simulink model "czasRegulacji_uchyb_przeregulowanie_simulink"  (R2025b)
settings: Solver=VariableStepAuto  StartTime=0.0  StopTime=20  RelTol=1e-3
settings Model: Creator=mefir  LastModifiedBy=mefir

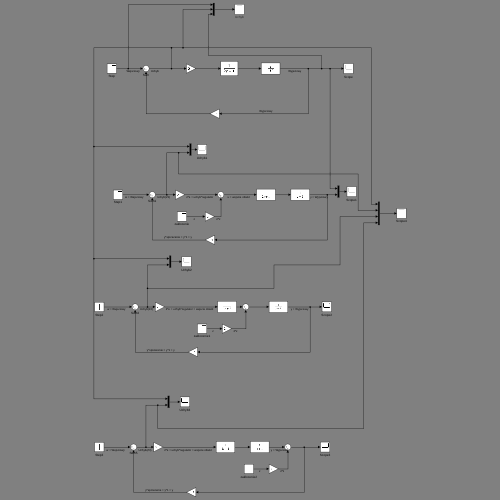
[thumbnail: Simulink's stored preview of the top-level diagram]
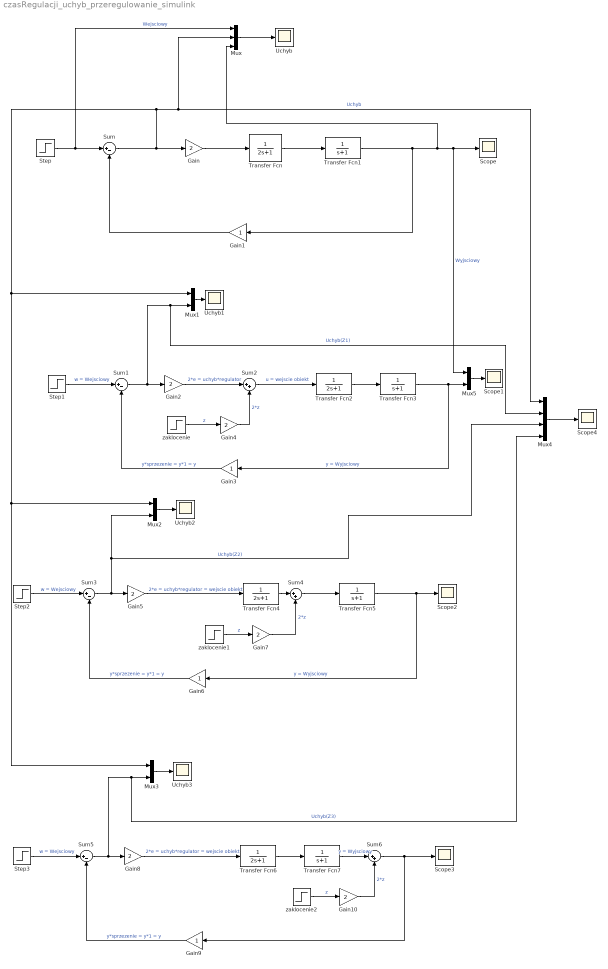
== system czasRegulacji_uchyb_przeregulowanie_simulink ==
  Gain{,2,4..5,7..8,10} (7 alike) : Gain  Gain=2
  Gain{1,3,6,9} (4 alike) : Gain
  Mux : Mux  Inputs=3
  Mux{1..3,5} (4 alike) : Mux  Inputs=2
  Mux4 : Mux
  Scope{,1..4} (5 alike) : Scope
      Scope settings: ActiveDisplayYMinimum=-0.06502980968093075  ActiveDisplayYMaximum=0.77577049871628523
      Scope1 settings: ActiveDisplayYMinimum=-0.023285806575956025  ActiveDisplayYMaximum=2.011000432811886  DataLoggingVariableName=ScopeData2
      Scope2 settings: ActiveDisplayYMinimum=-0.48841878311873588  ActiveDisplayYMaximum=2.237719338068338  DataLoggingVariableName=ScopeData4
      Scope3 settings: ActiveDisplayYMinimum=-0.61690021233914671  ActiveDisplayYMaximum=2.3886670662696021  DataLoggingVariableName=ScopeData6
      Scope4 settings: ActiveDisplayYMinimum=-1.25  ActiveDisplayYMaximum=1.25  DataLoggingVariableName=ScopeData8
  Step{,1..3} (4 alike) : Step  Time=0  SampleTime=0
  Sum{,1,3,5} (4 alike) : Sum  Inputs=|+-
  Sum2 : Sum  Inputs=|++
  Sum4 : Sum  Inputs=|++
  Sum6 : Sum  Inputs=|++
  Transfer Fcn{,2,4,6} (4 alike) : TransferFcn  Denominator=[2 1]
  Transfer Fcn{1,3,5,7} (4 alike) : TransferFcn  Denominator=[1 1]
  Uchyb{,1..3} (4 alike) : Scope
      Uchyb settings: ActiveDisplayYMinimum=-0.12499999999999997  ActiveDisplayYMaximum=1.125
      Uchyb1 settings: ActiveDisplayYMinimum=-0.62882694024493047  ActiveDisplayYMaximum=1.1809807711383256  DataLoggingVariableName=ScopeData3
      Uchyb2 settings: ActiveDisplayYMinimum=-0.62882694024493047  ActiveDisplayYMaximum=1.1809807711383256  DataLoggingVariableName=ScopeData5
      Uchyb3 settings: ActiveDisplayYMinimum=-0.70790013461355861  ActiveDisplayYMaximum=1.2874128671864817  DataLoggingVariableName=ScopeData7
  zaklocenie : Step  Time=0  SampleTime=0
  zaklocenie1 : Step  Time=0  SampleTime=0
  zaklocenie2 : Step  Time=0  SampleTime=0
  wires:
  Step/1 -> Mux/1, Sum/1  "Wejsciowy"
  Sum/1 -> Mux/2, Mux4/1, Mux3/1, Mux2/1, Mux1/1, Gain/1  "Uchyb"
  Gain/1 -> Transfer Fcn/1
  Transfer Fcn/1 -> Transfer Fcn1/1
  Transfer Fcn1/1 -> Mux/3, Mux5/1, Scope/1, Gain1/1  "Wyjsciowy"
  Gain1/1 -> Sum/2
  Mux/1 -> Uchyb/1
  Transfer Fcn3/1 -> Mux5/2, Gain3/1  "y = Wyjsciowy"
  Mux1/1 -> Uchyb1/1
  Gain3/1 -> Sum1/2  "y*sprzezenie = y*1 = y"
  Transfer Fcn2/1 -> Transfer Fcn3/1
  Step1/1 -> Sum1/1  "w = Wejsciowy"
  Sum1/1 -> Mux4/2, Mux1/2, Gain2/1  "Uchyb(Z1)"
  Gain2/1 -> Sum2/1  "2*e = uchyb*regulator"
  Sum2/1 -> Transfer Fcn2/1  "u = wejscie obiekt"
  zaklocenie/1 -> Gain4/1  "z"
  Gain4/1 -> Sum2/2  "2*z"
  Gain6/1 -> Sum3/2  "y*sprzezenie = y*1 = y"
  Step2/1 -> Sum3/1  "w = Wejsciowy"
  Transfer Fcn5/1 -> Scope2/1, Gain6/1  "y = Wyjsciowy"
  Sum3/1 -> Mux4/3, Mux2/2, Gain5/1  "Uchyb(Z2)"
  zaklocenie1/1 -> Gain7/1  "z"
  Gain7/1 -> Sum4/2  "2*z"
  Gain5/1 -> Transfer Fcn4/1  "2*e = uchyb*regulator = wejscie obiekt"
  Mux2/1 -> Uchyb2/1
  Transfer Fcn4/1 -> Sum4/1
  Sum4/1 -> Transfer Fcn5/1
  Gain9/1 -> Sum5/2  "y*sprzezenie = y*1 = y"
  Sum5/1 -> Mux4/4, Mux3/2, Gain8/1  "Uchyb(Z3)"
  Gain10/1 -> Sum6/2  "2*z"
  Mux3/1 -> Uchyb3/1
  zaklocenie2/1 -> Gain10/1  "z"
  Gain8/1 -> Transfer Fcn6/1  "2*e = uchyb*regulator = wejscie obiekt"
  Step3/1 -> Sum5/1  "w = Wejsciowy"
  Transfer Fcn6/1 -> Transfer Fcn7/1
  Transfer Fcn7/1 -> Sum6/1  "y = Wyjsciowy"
  Sum6/1 -> Gain9/1, Scope3/1
  Mux4/1 -> Scope4/1
  Mux5/1 -> Scope1/1
